simulink model "manning_test_system_nonlinear_test"  (R2022b)
settings: Solver=VariableStepAuto  StartTime=0.0  StopTime=5*N  RelTol=1e-3
undefined symbols (not defined in the file or in its folder): yd_ds
settings Model: Creator=chuan  LastModifiedBy=chuan

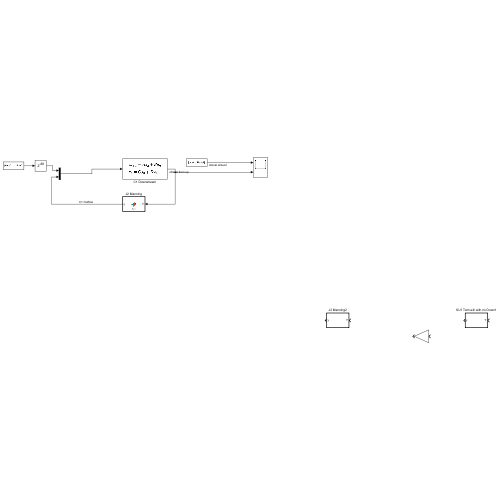
[thumbnail: Simulink's stored preview of the top-level diagram]
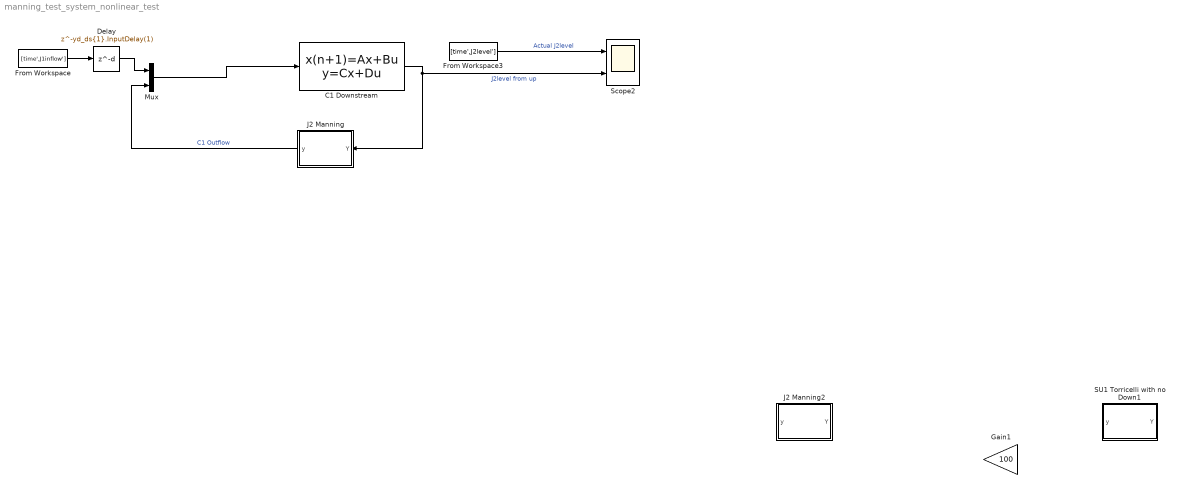
== system manning_test_system_nonlinear_test ==
  C1 Downstream : DiscreteStateSpace  A=yd_ds{1}.A  B=yd_ds{1}.B  C=yd_ds{1}.C  D=yd_ds{1}.D  SampleTime=yd_ds{1}.Ts
  Delay : Delay  DelayLength=yd_ds{1}.InputDelay(1)  InitialCondition=0
  From Workspace : FromWorkspace  VariableName=[time',J1inflow']
  From Workspace3 : FromWorkspace  VariableName=[time',J2level']
  Gain1 : Gain  Gain=100
  J2 Manning : MATLAB Function  TreatAsAtomicUnit=on
  J2 Manning2 : MATLAB Function  TreatAsAtomicUnit=on
  Mux : Mux  Inputs=2
  SU1 Torricelli with no Down1 : MATLAB Function  TreatAsAtomicUnit=on
  Scope2 : Scope  NumInputPorts=2
  wires:
  Mux/1 -> C1 Downstream/1
  J2 Manning/1(y) -> Mux/2  "C1 Outflow"
  From Workspace3/1 -> Scope2/1  "Actual J2level"
  C1 Downstream/1 -> J2 Manning/1(Y), Scope2/2  "J2level from up"
  From Workspace/1 -> Delay/1
  Delay/1 -> Mux/1

== matlab function manning_test_system_nonlinear_test/J2 Manning ==
  data: Y input; y output
function y = fcn(Y)
n = 0.015;
Sb = 0.0005;
B=8;
m = 1.5;

Y = max(Y,0);

y = (1/n)*(B*Y + m*Y.^2)*((B*Y + m*Y.^2)/(B + 2.*Y.*sqrt(1+m^2))).^(2/3) .* sqrt(Sb);

== matlab function manning_test_system_nonlinear_test/SU1 Torricelli with no Down1 ==
  data: Y input; y output
function y = fcn(Y)
Cd = 0.65;
A0 = 4;
g = 9.81;
Z0 = 9;
Yfull = 2;
H_star = Z0 + Yfull;

Y = max(Y,0);
H1 = Y + Z0;

if H1 >= H_star
    He = H1 - (Z0 + Yfull/2);
    y = Cd*A0*sqrt(2*g*He);
else
    CwL = (Cd*A0*sqrt(g))/(Yfull);
    y = CwL*(H1-Z0)^(1.5);
end

== matlab function manning_test_system_nonlinear_test/J2 Manning2 ==
  data: Y input; y output
function y = fcn(Y)
n = 0.015;
Sb = 0.0005;
B=8;
m = 1.5;

Y = max(Y,0);

y = (1/n)*(B*Y + m*Y.^2)*((B*Y + m*Y.^2)/(B + 2.*Y.*sqrt(1+m^2))).^(2/3) .* sqrt(Sb);
